simulink model "IPCBlockExampleTest"  (R2019a)
settings: Solver=VariableStepAuto  StartTime=0.0  StopTime=inf  RelTol=1e-3
settings Model: EnablePacing=on  Creator=wuyuanyi  LastModifiedBy=wuyua

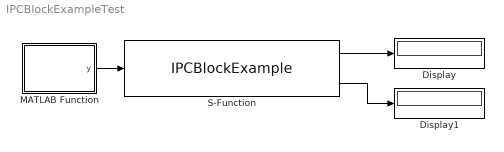
== system IPCBlockExampleTest ==
  Display : Display
  Display1 : Display
  MATLAB Function : MATLAB Function  TreatAsAtomicUnit=on
  S-Function : S-Function  FunctionName=IPCBlockExample  SFunctionDeploymentMode=off  EnableBusSupport=off
  wires:
  MATLAB Function/1(y) -> S-Function/1
  S-Function/1 -> Display/1
  S-Function/2 -> Display1/1

== matlab function IPCBlockExampleTest/MATLAB Function ==
  data: y output
function y = fcn()

y = rand(2,1);
